simulink model "Uklady_LTI_schemat_blokowy"  (R2022b)
settings: Solver=VariableStepAuto  StartTime=0.0  StopTime=10.0  RelTol=1e-3
model workspace (MAT data in the model file):
  F = 1000
  M = 1000
  a = 500
  c = 400
settings Model: Creator=Jakub  LastModifiedBy=Jakub

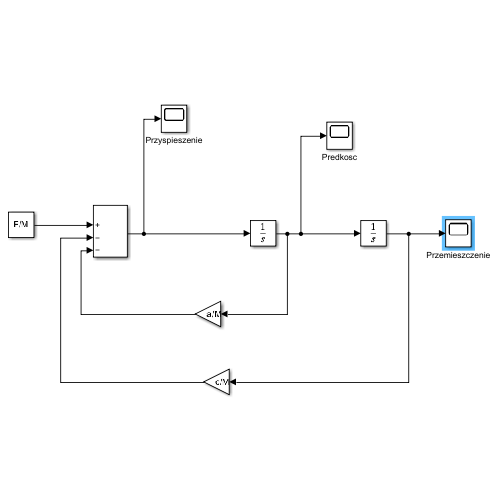
[thumbnail: Simulink's stored preview of the top-level diagram]
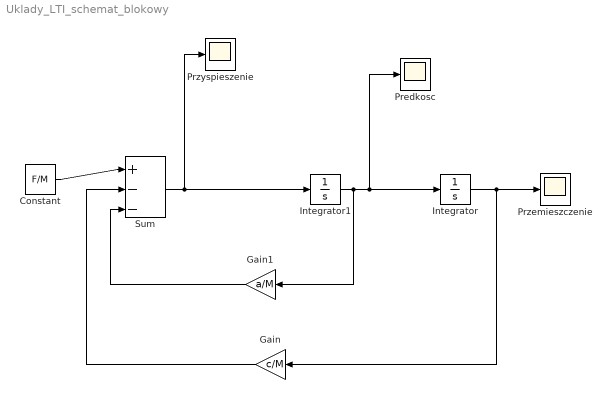
== system Uklady_LTI_schemat_blokowy ==
  Constant : Constant  Value=F/M
  Gain : Gain  Gain=c/M
  Gain1 : Gain  Gain=a/M
  Integrator : Integrator
  Integrator1 : Integrator
  Predkosc : Scope
  Przemieszczenie : Scope
  Przyspieszenie : Scope
  Sum : Sum  Inputs=|+--
  wires:
  Constant/1 -> Sum/1
  Gain1/1 -> Sum/3
  Gain/1 -> Sum/2
  Sum/1 -> Przyspieszenie/1, Integrator1/1
  Integrator1/1 -> Gain1/1, Predkosc/1, Integrator/1
  Integrator/1 -> Gain/1, Przemieszczenie/1
